simulink model "BMSSignals"  (R2018b)
settings: Solver=FixedStepAuto  StartTime=0.0  StopTime=10.0  RelTol=1e-3
settings Model: DataDictionary=Master_Dictionary.sldd  Creator=torni  LastModifiedBy=rubyg
settings RTWCC: SystemTargetFile=irt.tlc  TemplateMakefile=irt_default_tmf  Description=INTECRIO Real-Time Target
settings STFCustomTargetCC: TargetLangStandard=C99 (ISO)  CombineOutputUpdateFcns=on  MatFileLogging=on  SystemTargetFile=irt.tlc
settings GRTTargetCC: ParMdlRefBuildCompliant=off  CompOptLevelCompliant=off  ConcurrentExecutionCompliant=off  CPPClassGenCompliant=off  UseToolchainInfoCompliant=off

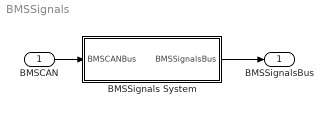
== system BMSSignals ==
  BMSCAN : Inport  OutDataTypeStr=Bus: CAN4Bus
  BMSSignals System : Subsystem
  BMSSignalsBus : Outport  OutDataTypeStr=Bus: BMSSignalsBus
  wires:
  BMSCAN/1 -> BMSSignals System/1(BMSCANBus)
  BMSSignals System/1(BMSSignalsBus) -> BMSSignalsBus/1

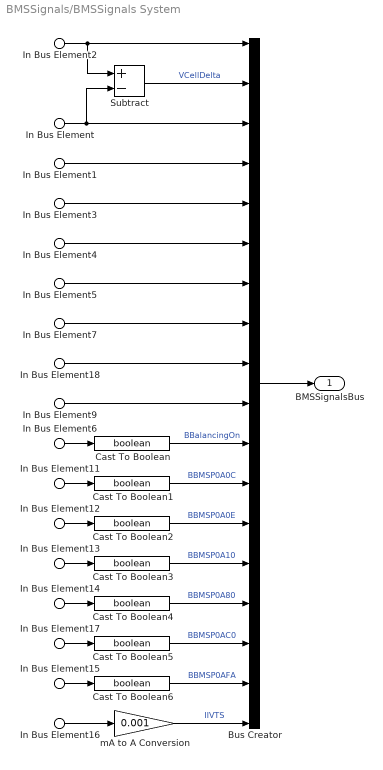
== system BMSSignals/BMSSignals System ==
  In Bus Element : Inport  PortName=BMSCANBus  Element=VCellMin
  In Bus Element1 : Inport  PortName=BMSCANBus  Element=VCellAverage
  In Bus Element2 : Inport  PortName=BMSCANBus  Element=VCellMax
  In Bus Element3 : Inport  PortName=BMSCANBus  Element=TCellMax
  In Bus Element4 : Inport  PortName=BMSCANBus  Element=NBMSDLC
  In Bus Element5 : Inport  PortName=BMSCANBus  Element=TCellMin
  In Bus Element7 : Inport  PortName=BMSCANBus  Element=IBMSHallEffect
  In Bus Element9 : Inport  PortName=BMSCANBus  Element=RCellAverage
  In Bus Element11 : Inport  PortName=BMSCANBus  Element=BBMSP0A0C
  In Bus Element12 : Inport  PortName=BMSCANBus  Element=BBMSP0A0E
  In Bus Element13 : Inport  PortName=BMSCANBus  Element=BBMSP0A10
  In Bus Element14 : Inport  PortName=BMSCANBus  Element=BBMSP0A80
  In Bus Element15 : Inport  PortName=BMSCANBus  Element=BBMSP0AFA
  In Bus Element16 : Inport  PortName=BMSCANBus  Element=IIVTS
  In Bus Element17 : Inport  PortName=BMSCANBus  Element=BBMSP0AC0
  In Bus Element18 : Inport  PortName=BMSCANBus  Element=VDCAccumulator
  In Bus Element6 : Inport  PortName=BMSCANBus  Element=BBalancingOn
  Bus Creator : BusCreator  Inputs=18  OutDataTypeStr=Bus: BMSSignalsBus
  Cast To Boolean{,1..6} (7 alike) : DataTypeConversion  OutDataTypeStr=boolean
  Subtract : Sum  Inputs=+-
  mA to A Conversion : Gain  Gain=0.001
  BMSSignalsBus : Outport  OutDataTypeStr=Bus: BMSSignalsBus
  wires:
  Bus Creator/1 -> BMSSignalsBus/1
  In Bus Element/1 -> Bus Creator/3, Subtract/2
  In Bus Element1/1 -> Bus Creator/4
  In Bus Element2/1 -> Bus Creator/1, Subtract/1
  In Bus Element3/1 -> Bus Creator/5
  In Bus Element4/1 -> Bus Creator/6
  In Bus Element5/1 -> Bus Creator/7
  In Bus Element7/1 -> Bus Creator/8
  In Bus Element18/1 -> Bus Creator/9
  In Bus Element9/1 -> Bus Creator/10
  In Bus Element6/1 -> Cast To Boolean/1
  In Bus Element11/1 -> Cast To Boolean1/1
  In Bus Element12/1 -> Cast To Boolean2/1
  In Bus Element13/1 -> Cast To Boolean3/1
  In Bus Element14/1 -> Cast To Boolean4/1
  In Bus Element16/1 -> mA to A Conversion/1
  In Bus Element17/1 -> Cast To Boolean5/1
  Subtract/1 -> Bus Creator/2  "VCellDelta"
  mA to A Conversion/1 -> Bus Creator/18  "IIVTS"
  In Bus Element15/1 -> Cast To Boolean6/1
  Cast To Boolean/1 -> Bus Creator/11  "BBalancingOn"
  Cast To Boolean1/1 -> Bus Creator/12  "BBMSP0A0C"
  Cast To Boolean2/1 -> Bus Creator/13  "BBMSP0A0E"
  Cast To Boolean3/1 -> Bus Creator/14  "BBMSP0A10"
  Cast To Boolean4/1 -> Bus Creator/15  "BBMSP0A80"
  Cast To Boolean5/1 -> Bus Creator/16  "BBMSP0AC0"
  Cast To Boolean6/1 -> Bus Creator/17  "BBMSP0AFA"
